simulink model "BAppsOK"  (R2024b)
settings: configuration reference "STM32H7_Config" (kept outside this file)
undefined symbols (not defined in the file): pAppsBrakeThreshold, pAppsThrottleThreshold, tSystemsTask
libraries: simulink x2
settings Model: DataDictionary=Master_Dictionary.sldd  EnableAccessToBaseWorkspace=off  Creator=torni  LastModifiedBy=Will
settings ConfigSetRef: SourceName=STM32H7_Config

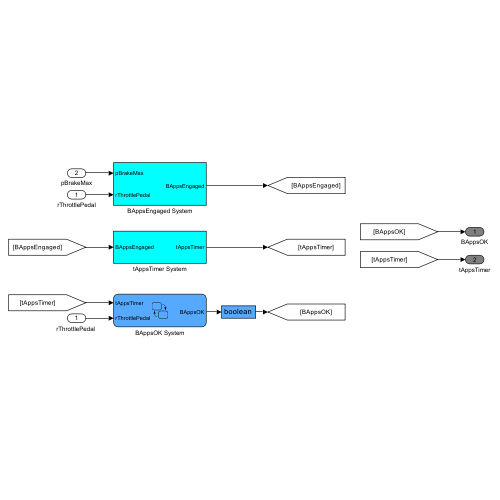
[thumbnail: Simulink's stored preview of the top-level diagram]
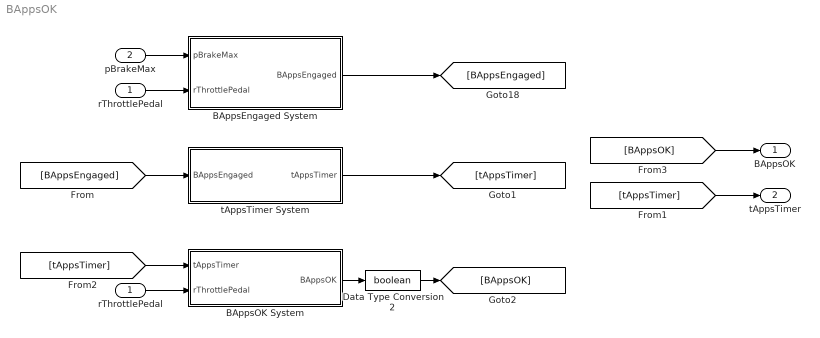
== system BAppsOK ==
  rThrottlePedal : Inport  OutDataTypeStr=double
  pBrakeMax : Inport  Port=2  OutDataTypeStr=double
  BAppsEngaged System : Subsystem
  BAppsOK System : Stateflow chart  TreatAsAtomicUnit=on
  Data Type Conversion2 : DataTypeConversion  OutDataTypeStr=boolean  SaturateOnIntegerOverflow=off  RndMeth=Floor
  "rThrottlePedal " : InportShadow  OutDataTypeStr=double
  tAppsTimer System : Subsystem
  BAppsOK : Outport  OutDataTypeStr=boolean  VectorParamsAs1DForOutWhenUnconnected=off
  tAppsTimer : Outport  Port=2  OutDataTypeStr=double  VectorParamsAs1DForOutWhenUnconnected=off
  wires:
  rThrottlePedal/1 -> BAppsEngaged System/2(rThrottlePedal)
  pBrakeMax/1 -> BAppsEngaged System/1(pBrakeMax)
  BAppsEngaged System/1(BAppsEngaged) -> [BAppsEngaged]
  [BAppsEngaged] -> tAppsTimer System/1(BAppsEngaged)
  tAppsTimer System/1(tAppsTimer) -> [tAppsTimer]
  [tAppsTimer] -> tAppsTimer/1
  [tAppsTimer] -> BAppsOK System/1(tAppsTimer)
  "rThrottlePedal "/1 -> BAppsOK System/2(rThrottlePedal)
  [BAppsOK] -> BAppsOK/1
  BAppsOK System/1(BAppsOK) -> Data Type Conversion2/1
  Data Type Conversion2/1 -> [BAppsOK]

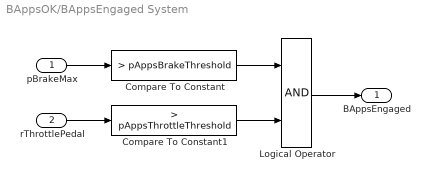
== system BAppsOK/BAppsEngaged System ==
  pBrakeMax : Inport  OutDataTypeStr=double
  rThrottlePedal : Inport  Port=2  OutDataTypeStr=double
  Compare To Constant : simulink/Logic and Bit Operations/Compare To Constant  relop=>  const=pAppsBrakeThreshold  OutDataTypeStr=boolean
  Compare To Constant1 : simulink/Logic and Bit Operations/Compare To Constant  relop=>  const=pAppsThrottleThreshold  OutDataTypeStr=boolean
  Logical Operator : Logic  AllPortsSameDT=off  OutDataTypeStr=boolean
  BAppsEngaged : Outport  OutDataTypeStr=boolean  VectorParamsAs1DForOutWhenUnconnected=off
  wires:
  pBrakeMax/1 -> Compare To Constant/1
  Compare To Constant/1 -> Logical Operator/1
  Compare To Constant1/1 -> Logical Operator/2
  Logical Operator/1 -> BAppsEngaged/1
  rThrottlePedal/1 -> Compare To Constant1/1

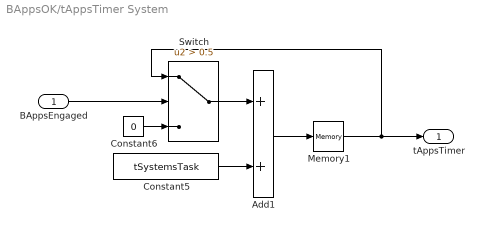
== system BAppsOK/tAppsTimer System ==
  BAppsEngaged : Inport  OutDataTypeStr=boolean
  Add1 : Sum
  Constant5 : Constant  Value=tSystemsTask
  Constant6 : Constant  Value=0
  Memory1 : Memory  InheritSampleTime=on
  Switch : Switch  Criteria=u2 > Threshold  Threshold=0.5  SaturateOnIntegerOverflow=off  InputSameDT=off
  tAppsTimer : Outport  OutDataTypeStr=double  VectorParamsAs1DForOutWhenUnconnected=off
  wires:
  Add1/1 -> Memory1/1
  Memory1/1 -> Switch/1, tAppsTimer/1
  Switch/1 -> Add1/1
  Constant5/1 -> Add1/2
  Constant6/1 -> Switch/3
  BAppsEngaged/1 -> Switch/2

== stateflow chart BAppsOK/BAppsOK System ==
  state Entrance
    BAppsOK = 1;
  state Reset
    BAppsOK = 0;
  Entrance -> Reset : [tAppsTimer > 0.5]
  (default) -> Entrance
  Reset -> Entrance : [rThrottlePedal < 6.25]
  data: tAppsTimer input; BAppsOK output; rThrottlePedal input
